simulink model "EKF"  (R2020b)
settings: Solver=VariableStepAuto  StartTime=0.0  StopTime=10.0  RelTol=1e-3
settings Model: Creator=ST  LastModifiedBy=ST

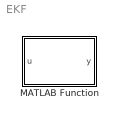
== system EKF ==
  MATLAB Function : MATLAB Function  TreatAsAtomicUnit=on

== matlab function EKF/MATLAB Function ==
  data: u input; y output
function y = fcn(u)

y = u;
